simulink subsystem "ChillerNoCoolant"  (R2024b)
settings: Solver=VariableStepAuto  StartTime=0.0  StopTime=10.0  RelTol=1e-3
undefined symbols (not defined in the file or in its folder): chiller
libraries: fl_lib x13, nesl_utility x3, simulink x1
settings Model: Creator=jjha  LastModifiedBy=jjha

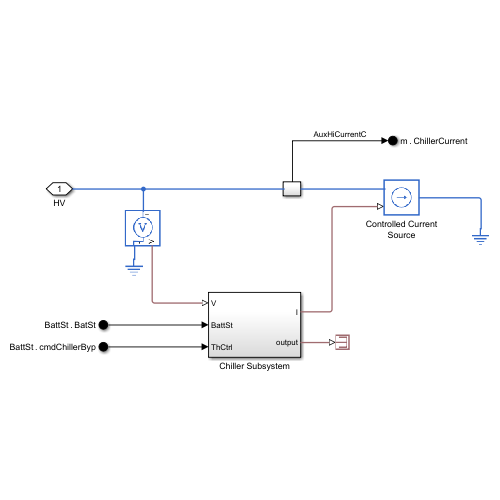
[thumbnail: Simulink's stored preview of the top-level diagram]
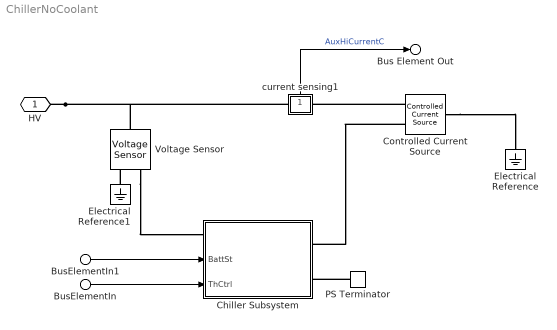
== system ChillerNoCoolant ==
  BusElementIn : Inport  PortName=BattSt  Element=cmdChillerByp
  BusElementIn1 : Inport  PortName=BattSt  Element=BatSt
  Chiller Subsystem : Subsystem
      settings: PortSchema="{\"entries\":[{\"content\":{\"sides\":[{\"content\":{\"connectorIds\":[\"LConn1\",\"In1\",\"In2\"]},\"type\":\"ConnectorPlacement.EquallySpacedRectSide\",\"uuid\":\"d995acd0-973b-4873-b050-eaa71c2c53f5\"},{\"content\":{\"connectorIds\":[\"RConn1\",\"RConn2\"],\"side\":\"RIGHT\"},\"type\":\"ConnectorPlacement.EquallySpacedRectSide\",\"uuid\":\"f40dc2d9-a9a2-427c-8e3f-65ba63c73559\"},{\"content\":{\"connectorIds\":[],\"side\":\"TOP\"},\"type\":\"ConnectorPlacement.EquallySpacedRectSide\",\"uuid\":\"1868aaf5-b9f5-4fdb-94e9-4b9189d403a5\"}]},\"type\":\"ConnectorPlacement.EquallySpacedConnector\",\"uuid\":\"c13a0ccf-549d-47cf-8e66-a96ce55255c8\"}],\"packageUris\":[\"http://schema.mathworks.com/mf0/Connector/R2020b\"],\"version\":\"1.0\"}"
  Controlled Current Source : fl_lib/Electrical/Electrical Sources/Controlled Current Source
  Electrical Reference : fl_lib/Electrical/Electrical Elements/Electrical Reference
  Electrical Reference1 : fl_lib/Electrical/Electrical Elements/Electrical Reference
  PS Terminator : fl_lib/Physical Signals/Sinks/PS Terminator
  Voltage Sensor : fl_lib/Electrical/Electrical Sensors/Voltage Sensor
  current sensing1 : Subsystem
      settings: PortSchema="{\"entries\":[{\"content\":{\"sides\":[{\"content\":{\"connectorIds\":[\"LConn1\"]},\"type\":\"ConnectorPlacement.EquallySpacedRectSide\",\"uuid\":\"be2815b5-7c4b-4452-9f46-9765620d338b\"},{\"content\":{\"connectorIds\":[\"RConn1\"],\"side\":\"RIGHT\"},\"type\":\"ConnectorPlacement.EquallySpacedRectSide\",\"uuid\":\"398ebab2-f4fa-4d00-bf6e-74bf1f6972c5\"},{\"content\":{\"connectorIds\":[\"Out1\"],\"side\":\"TOP\"},\"type\":\"ConnectorPlacement.EquallySpacedRectSide\",\"uuid\":\"f18d5713-17ec-4be9-9072-3e03c5a4f599\"}]},\"type\":\"ConnectorPlacement.EquallySpacedConnector\",\"uuid\":\"966ec05e-6316-4039-8e26-1d6b096cf423\"}],\"packageUris\":[\"http://schema.mathworks.com/mf0/Connector/R2020b\"],\"version\":\"1.0\"}"
  HV : PMIOPort  Side=Left
  Bus Element Out : Outport  PortName=m  Element=ChillerCurrent
  wires:
  current sensing1/1("   ") -> Bus Element Out/1  "AuxHiCurrentC"
  BusElementIn/1 -> Chiller Subsystem/2(ThCtrl)
  BusElementIn1/1 -> Chiller Subsystem/1(BattSt)
  connections:
  HV/RConn1 -- current sensing1/LConn1 -- Voltage Sensor/LConn1
  Voltage Sensor/RConn1 -- Chiller Subsystem/LConn1
  Electrical Reference1/LConn1 -- Voltage Sensor/RConn2
  Controlled Current Source/RConn1 -- Chiller Subsystem/RConn1
  Controlled Current Source/LConn1 -- Electrical Reference/LConn1
  Controlled Current Source/RConn2 -- current sensing1/RConn1
  PS Terminator/LConn1 -- Chiller Subsystem/RConn2

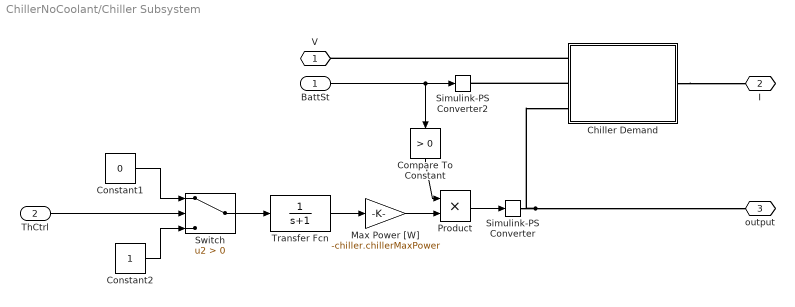
== system ChillerNoCoolant/Chiller Subsystem ==
  BattSt : Inport
  ThCtrl : Inport  Port=2
  Chiller Demand : Subsystem
  Compare To Constant : simulink/Logic and Bit Operations/Compare To Constant  relop=>  const=0  OutDataTypeStr=boolean
  Constant1 : Constant  Value=0
  Constant2 : Constant
  Max Power [W] : Gain  Gain=-chiller.chillerMaxPower
  Product : Product
  Simulink-PS Converter : nesl_utility/Simulink-PS Converter  PhysicalDomain=network_engine_domain  SubClassName=ps_input  LeftPortType=input  RightPortType=output  PseudoPeriodic=off  Frequencies=[]  NoiseDistribution=none  NoiseParameters=[]  Unit=W  AffineConversion=off  FilteringAndDerivatives=provide  SimscapeFilterOrder=1  InputFilterTimeConstant=0.001  UdotUserProvided=0
  Simulink-PS Converter2 : nesl_utility/Simulink-PS Converter  PhysicalDomain=network_engine_domain  SubClassName=ps_input  LeftPortType=input  RightPortType=output  PseudoPeriodic=off  Frequencies=[]  NoiseDistribution=none  NoiseParameters=[]  Unit=1  AffineConversion=off  FilteringAndDerivatives=provide  SimscapeFilterOrder=1  InputFilterTimeConstant=0.001  UdotUserProvided=0
  Switch : Switch  Criteria=u2 > Threshold  SaturateOnIntegerOverflow=off  InputSameDT=off
  Transfer Fcn : TransferFcn  Denominator=[1 1]
  V : PMIOPort  Side=Left
  I : PMIOPort  Port=2  Side=Right
  output : PMIOPort  Port=3  Side=Right
  wires:
  Max Power [W]/1 -> Product/2
  Switch/1 -> Transfer Fcn/1
  ThCtrl/1 -> Switch/2
  Transfer Fcn/1 -> Max Power [W]/1
  BattSt/1 -> Compare To Constant/1, Simulink-PS Converter2/1
  Product/1 -> Simulink-PS Converter/1
  Compare To Constant/1 -> Product/1
  Constant2/1 -> Switch/3
  Constant1/1 -> Switch/1
  connections:
  Simulink-PS Converter/RConn1 -- output/RConn1 -- Chiller Demand/LConn3
  Chiller Demand/LConn1 -- V/RConn1
  Chiller Demand/LConn2 -- Simulink-PS Converter2/RConn1
  Chiller Demand/RConn1 -- I/RConn1

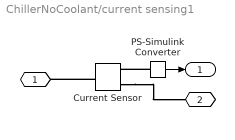
== system ChillerNoCoolant/current sensing1 ==
  Current Sensor : fl_lib/Electrical/Electrical Sensors/Current Sensor
  PS-Simulink Converter : nesl_utility/PS-Simulink Converter  PhysicalDomain=network_engine_domain  SubClassName=ps_output  LeftPortType=input  RightPortType=output  PseudoPeriodic=off  Frequencies=[]  VectorFormat=inherit  Unit=inherit  AffineConversion=off
  "  " : PMIOPort  Side=Left
  " " : PMIOPort  Port=2  Side=Right
  "   " : Outport
  wires:
  PS-Simulink Converter/1 -> "   "/1
  connections:
  PS-Simulink Converter/LConn1 -- Current Sensor/RConn1
  Current Sensor/LConn1 -- "  "/RConn1
  Current Sensor/RConn2 -- " "/RConn1

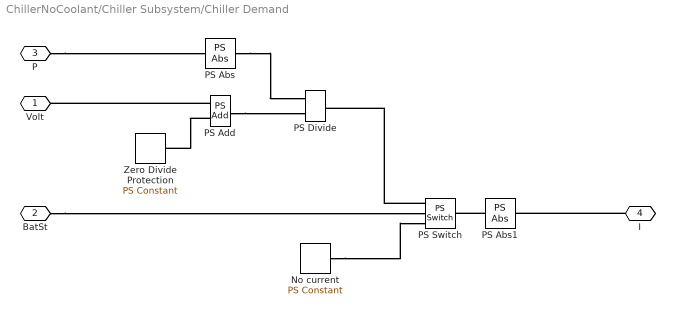
== system ChillerNoCoolant/Chiller Subsystem/Chiller Demand ==
  No current : fl_lib/Physical Signals/Sources/PS Constant  constant=0 A
  PS Abs : fl_lib/Physical Signals/Nonlinear Operators/PS Abs
      settings: InternalSimscapePortConfiguration="{\"Bottom\":[],\"Left\":[{\"id\":\"I\",\"label\":\"\",\"type\":\"input\"}],\"Right\":[{\"id\":\"O\",\"label\":\"\",\"type\":\"output\"}],\"Top\":[]}"
  PS Abs1 : fl_lib/Physical Signals/Nonlinear Operators/PS Abs
      settings: InternalSimscapePortConfiguration="{\"Bottom\":[],\"Left\":[{\"id\":\"I\",\"label\":\"\",\"type\":\"input\"}],\"Right\":[{\"id\":\"O\",\"label\":\"\",\"type\":\"output\"}],\"Top\":[]}"
  PS Add : fl_lib/Physical Signals/Functions/PS Add
  PS Divide : fl_lib/Physical Signals/Functions/PS Divide
  PS Switch : fl_lib/Physical Signals/Nonlinear Operators/PS Switch  Threshold=0.5
      settings: InternalSimscapePortConfiguration="{\"Bottom\":[],\"Left\":[{\"id\":\"I1\",\"label\":\"\",\"type\":\"input\"},{\"id\":\"I2\",\"label\":\"\",\"type\":\"input\"},{\"id\":\"I3\",\"label\":\"\",\"type\":\"input\"}],\"Right\":[{\"id\":\"O\",\"label\":\"\",\"type\":\"output\"}],\"Top\":[]}"
  Zero Divide Protection : fl_lib/Physical Signals/Sources/PS Constant  constant=1 V
  Volt : PMIOPort  Side=Left
  BatSt : PMIOPort  Port=2  Side=Left
  P : PMIOPort  Port=3  Side=Left
  I : PMIOPort  Port=4  Side=Right
  connections:
  No current/RConn1 -- PS Switch/LConn3
  PS Add/LConn1 -- Volt/RConn1
  PS Switch/LConn1 -- PS Divide/RConn1
  BatSt/RConn1 -- PS Switch/LConn2
  I/RConn1 -- PS Abs1/RConn1
  PS Add/RConn1 -- PS Divide/LConn2
  PS Add/LConn2 -- Zero Divide Protection/RConn1
  PS Abs/RConn1 -- PS Divide/LConn1
  P/RConn1 -- PS Abs/LConn1
  PS Abs1/LConn1 -- PS Switch/RConn1
